simulink library "discreteGainScheduledFilteredPID"  (R2022a)
settings: Solver=VariableStepAuto  StartTime=0.0  StopTime=10.0  RelTol=1e-3
undefined symbols (not defined in the file): Ts
libraries: discreteFilter_ul x1
settings Model: Creator=adabney  LastModifiedBy=adabney

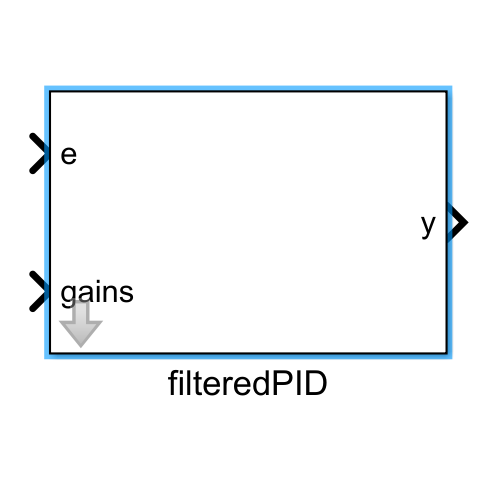
[thumbnail: Simulink's stored preview of the top-level diagram]
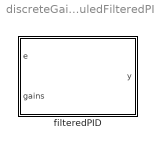
== system discreteGainScheduledFilteredPID ==
  filteredPID : Subsystem  mask{tau=0, Ts=Ts}
      mask prompts: tau "Filter Time Constant"; Ts "Sample Time"
      mask DialogControl DescTextVar Prompt: Gain-scheduled Discrete-time Filtered-PID Controller
      mask DialogControl ParameterGroupVar Prompt: Controller Inputs

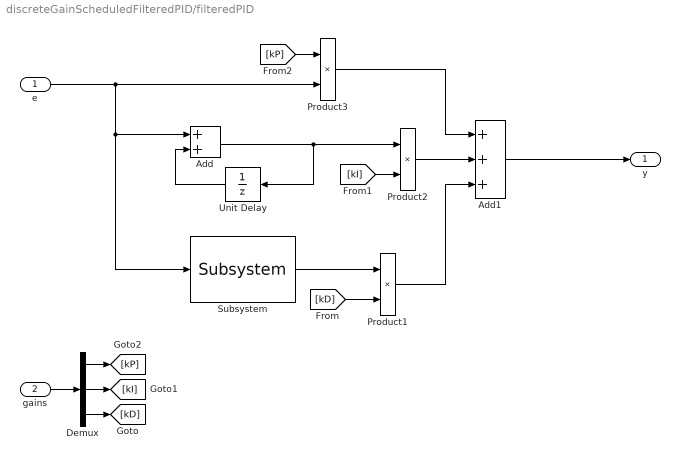
== system discreteGainScheduledFilteredPID/filteredPID ==
  e : Inport
  gains : Inport  Port=2
  Add : Sum
  Add1 : Sum  Inputs=+++
  Demux : Demux  Outputs=3
  Product1 : Product
  Product2 : Product
  Product3 : Product
  Subsystem : discreteFilter_ul/Subsystem  Ts=Ts  tau=tau
  Unit Delay : UnitDelay  SampleTime=-1  HasFrameUpgradeWarning=on
  y : Outport
  wires:
  Product1/1 -> Add1/3
  Add/1 -> Product2/1, Unit Delay/1
  Product3/1 -> Add1/1
  e/1 -> Product3/2, Subsystem/1, Add/1
  [kD] -> Product1/2
  [kI] -> Product2/2
  [kP] -> Product3/1
  Add1/1 -> y/1
  Product2/1 -> Add1/2
  Unit Delay/1 -> Add/2
  Subsystem/1 -> Product1/1
  gains/1 -> Demux/1
  Demux/1 -> [kP]
  Demux/2 -> [kI]
  Demux/3 -> [kD]
